simulink model "LinksVDCR1"  (R2020b)
settings: Solver=ode45  StartTime=0.0  StopTime=20  FixedStep=0.001  RelTol=1e-5  AbsTol=1e-5
undefined symbols (not defined in the file or in its folder): X, Y, Z
libraries: sm_lib x18, nesl_utility x9
settings Model: Creator=liikaneh  LastModifiedBy=humaloja
settings SolverCC: ZeroCrossAlgorithm=Adaptive  AlgebraicLoopSolver=LineSearch
settings DataIOCC: ReturnWorkspaceOutputs=off
settings DebuggingCC: ArithmeticOperatorsInVariantConditions=warning
settings SFSimCC: SimUseLocalCustomCode=off  CustomCodeUndefinedFunction=UseInterfaceOnly
settings RTWCC: RTWUseLocalCustomCode=off

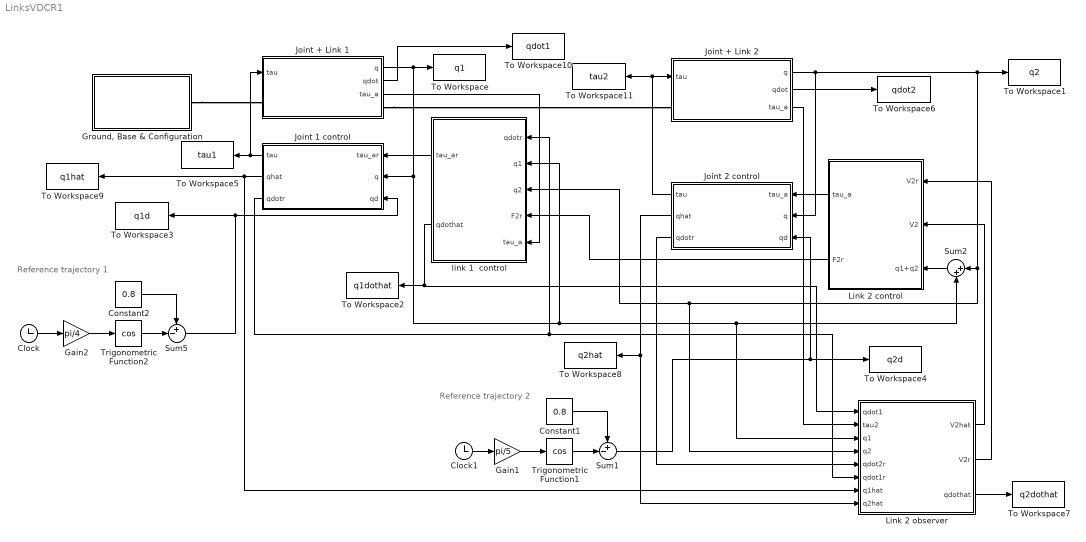
== system LinksVDCR1 ==
  note: Reference trajectory 1
  note: Reference trajectory 2
  Clock : Clock
  Clock1 : Clock
  Constant1 : Constant  Value=0.8
  Constant2 : Constant  Value=0.8
  Gain1 : Gain  Gain=pi/5
  Gain2 : Gain  Gain=pi/4
  "Ground, Base & Configuration" : Subsystem
  Joint + Link 1 : Subsystem
  Joint + Link 2 : Subsystem
  Joint 1 control : Subsystem
  Joint 2 control : Subsystem
  Link 2 control : Subsystem
  Link 2 observer : Subsystem
  Sum1 : Sum  Inputs=+-|
  Sum2 : Sum  Inputs=|++
  Sum5 : Sum  Inputs=+-|
  To Workspace : ToWorkspace  VariableName=q1  SaveFormat=Timeseries  SampleTime=-1
  To Workspace1 : ToWorkspace  VariableName=q2  SaveFormat=Timeseries  SampleTime=-1
  To Workspace10 : ToWorkspace  VariableName=qdot1  SaveFormat=Timeseries  SampleTime=-1
  To Workspace11 : ToWorkspace  VariableName=tau2  SaveFormat=Timeseries  SampleTime=-1
  To Workspace2 : ToWorkspace  VariableName=q1dothat  SaveFormat=Timeseries  SampleTime=-1
  To Workspace3 : ToWorkspace  VariableName=q1d  SaveFormat=Timeseries  SampleTime=-1
  To Workspace4 : ToWorkspace  VariableName=q2d  SaveFormat=Timeseries  SampleTime=-1
  To Workspace5 : ToWorkspace  VariableName=tau1  SaveFormat=Timeseries  SampleTime=-1
  To Workspace6 : ToWorkspace  VariableName=qdot2  SaveFormat=Timeseries  SampleTime=-1
  To Workspace7 : ToWorkspace  VariableName=q2dothat  SaveFormat=Timeseries  SampleTime=-1
  To Workspace8 : ToWorkspace  VariableName=q2hat  SaveFormat=Timeseries  SampleTime=-1
  To Workspace9 : ToWorkspace  VariableName=q1hat  SaveFormat=Timeseries  SampleTime=-1
  Trigonometric Function1 : Trigonometry  Operator=cos
  Trigonometric Function2 : Trigonometry  Operator=cos
  link 1  control : Subsystem
  wires:
  Joint + Link 1/1(q) -> To Workspace/1, link 1  control/2(q1), Link 2 observer/3(q1), Sum2/2, Joint 1 control/2(q)
  Constant1/1 -> Sum1/1
  Joint + Link 2/1(q) -> Joint 2 control/2(q), link 1  control/3(q2), Link 2 observer/4(q2), Sum2/1, To Workspace1/1
  Sum2/1 -> Link 2 control/3(q1+q2)
  Link 2 observer/1(V2hat) -> Link 2 control/2(V2)
  Link 2 observer/2(V2r) -> Link 2 control/1(V2r)
  Clock1/1 -> Gain1/1
  Gain1/1 -> Trigonometric Function1/1
  Sum5/1 -> To Workspace3/1, Joint 1 control/3(qd)
  Sum1/1 -> Joint 2 control/3(qd), To Workspace4/1
  Constant2/1 -> Sum5/1
  Gain2/1 -> Trigonometric Function2/1
  Clock/1 -> Gain2/1
  Link 2 control/1(tau_a) -> Joint 2 control/1(tau_a)
  Joint 1 control/1(tau) -> Joint + Link 1/1(tau), To Workspace5/1
  Joint + Link 2/3(tau_a) -> Link 2 observer/2(tau2)
  Joint + Link 1/3(tau_a) -> link 1  control/5(tau_a)
  Joint 1 control/2(qhat) -> To Workspace9/1, Link 2 observer/7(q1hat)
  Joint 1 control/3(qdotr) -> Link 2 observer/6(qdot1r), link 1  control/1(qdotr)
  link 1  control/1(tau_ar) -> Joint 1 control/1(tau_ar)
  Link 2 control/2(F2r) -> link 1  control/4(F2r)
  Trigonometric Function1/1 -> Sum1/2
  Trigonometric Function2/1 -> Sum5/2
  Joint 2 control/1(tau) -> Joint + Link 2/1(tau), To Workspace11/1
  Joint 2 control/2(qhat) -> Link 2 observer/8(q2hat), To Workspace8/1
  Joint 2 control/3(qdotr) -> Link 2 observer/5(qdot2r)
  Joint + Link 1/2(qdot) -> To Workspace10/1
  Joint + Link 2/2(qdot) -> To Workspace6/1
  link 1  control/2(qdothat) -> Link 2 observer/1(qdot1), To Workspace2/1
  Link 2 observer/3(qdothat) -> To Workspace7/1
  connections:
  "Ground, Base & Configuration"/RConn1 -- Joint + Link 1/LConn1
  Joint + Link 1/RConn1 -- Joint + Link 2/LConn1

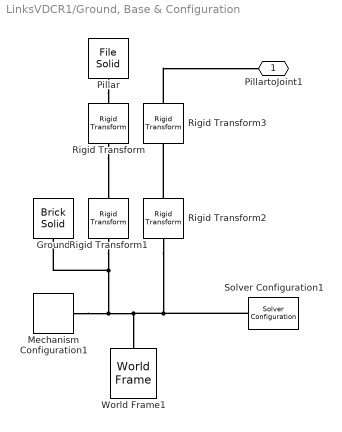
== system LinksVDCR1/Ground, Base & Configuration ==
  Ground : sm_lib/Body Elements/Brick Solid  GraphicAmbientColor=[0.15 0.15 0.15 1.0]  BasedOnType=Density  BrickDimensions=[1 1 0.05]  BrickDimensionUnits=m  CenterOfMass=[0 0 0]  CenterOfMassUnits=m  GraphicDiffuseColor=[0.2 0.2 0.2]  Density=1000  DensityUnits=kg/m^3  DoExposeReferenceFrame=on  GraphicEmissiveColor=[0.0 0.0 0.0 1.0]  ExportEntireGeometry=off  SerializedFrames=<Frames/>  MarkerShape=Sphere  MarkerSize=10  GraphicType=FromGeometry  InertiaType=CalculateFromGeometry  Mass=1  MassUnits=kg  MomentsOfInertia=[1 1 1]  MomentsOfInertiaUnits=kg*m^2  GraphicOpacity=1.0  ProductsOfInertia=[1 1 1]  ProductsOfInertiaUnits=kg*m^2  GraphicShininess=75  GraphicSpecularColor=[0.5 0.5 0.5 1.0]  GraphicVisPropType=SimpleVisualProperties
  Mechanism Configuration1 : sm_lib/Utilities/Mechanism Configuration  UniformGravity=Constant  GravityVector=[0 0 -9.80655]  GravityVectorUnits=m/s^2  GravityUnits=m/s^2  LinearizationDelta=0.002  JointModeTransitionNonlinearIterations=2
  Pillar : sm_lib/Body Elements/File Solid  ExtGeomFileName=Base.STEP  UnitType=FromFile  ExtGeomFileUnits=m  StepReaderType=OCC  ExportConvexHullGeometry=off  InertiaType=CalculateFromGeometry  Mass=1  MassUnits=kg  CenterOfMass=[0 0 0]  CenterOfMassUnits=m  MomentsOfInertia=[1 1 1]  MomentsOfInertiaUnits=kg*m^2  ProductsOfInertia=[1 1 1]  ProductsOfInertiaUnits=kg*m^2  BasedOnType=Density  Density=1000  DensityUnits=kg/m^3  DoExposeReferenceFrame=on  SerializedFrames=<Frames/>  GraphicType=FromGeometry  MarkerShape=Sphere  MarkerSize=10  GraphicVisPropType=SimpleVisualProperties  GraphicDiffuseColor=[0.2 0.2 0.2]  GraphicSpecularColor=[0.5 0.5 0.5 1.0]  GraphicAmbientColor=[0.15 0.15 0.15 1.0]  GraphicEmissiveColor=[0.0 0.0 0.0 1.0]  GraphicShininess=75  GraphicOpacity=1.0
  Rigid Transform : sm_lib/Frames and Transforms/Rigid Transform  TranslationMethod=None  TranslationStandardOffset=0  TranslationLengthUnit=m  TranslationStandardAxis=+Z  TranslationCartesianOffset=[0 0 0]  TranslationROffset=0  TranslationROffsetUnits=m  TranslationZOffset=0  TranslationZOffsetUnits=m  TranslationThetaOffset=0  TranslationThetaOffsetUnits=deg  RotationMethod=StandardAxis  RotationAngleUnits=deg  RotationStandardAxis=+Y  RotationAngle=180  RotationArbitraryAxis=[0 0 1]  FollAlignAxisA=+X  BaseAlignAxisA=+Y  FollAlignAxisB=+Y  BaseAlignAxisB=+Z  RotationSequenceAxes=FollowerAxes  RotationSequence=XYX  RotationSequenceAngles=[0 0 0]  RotationSequenceAnglesUnits=deg  RotationMatrix=[1 0 0; 0 1 0; 0 0 1]
  Rigid Transform1 : sm_lib/Frames and Transforms/Rigid Transform  TranslationMethod=None  TranslationStandardOffset=0  TranslationLengthUnit=m  TranslationStandardAxis=+Z  TranslationCartesianOffset=[0 0 0]  TranslationROffset=0  TranslationROffsetUnits=m  TranslationZOffset=0  TranslationZOffsetUnits=m  TranslationThetaOffset=0  TranslationThetaOffsetUnits=deg  RotationMethod=StandardAxis  RotationAngleUnits=deg  RotationStandardAxis=+Z  RotationAngle=90  RotationArbitraryAxis=[0 0 1]  FollAlignAxisA=+X  BaseAlignAxisA=+Y  FollAlignAxisB=+Y  BaseAlignAxisB=+Z  RotationSequenceAxes=FollowerAxes  RotationSequence=XYX  RotationSequenceAngles=[0 0 0]  RotationSequenceAnglesUnits=deg  RotationMatrix=[1 0 0; 0 1 0; 0 0 1]
  Rigid Transform2 : sm_lib/Frames and Transforms/Rigid Transform  TranslationMethod=StandardAxis  TranslationStandardOffset=0.470  TranslationLengthUnit=m  TranslationStandardAxis=+Z  TranslationCartesianOffset=[0 0 0]  TranslationROffset=0  TranslationROffsetUnits=m  TranslationZOffset=0  TranslationZOffsetUnits=m  TranslationThetaOffset=0  TranslationThetaOffsetUnits=deg  RotationMethod=None  RotationAngleUnits=deg  RotationStandardAxis=+Z  RotationAngle=0.0  RotationArbitraryAxis=[0 0 1]  FollAlignAxisA=+X  BaseAlignAxisA=+Y  FollAlignAxisB=+Y  BaseAlignAxisB=+Z  RotationSequenceAxes=FollowerAxes  RotationSequence=XYX  RotationSequenceAngles=[0 0 0]  RotationSequenceAnglesUnits=deg  RotationMatrix=[1 0 0; 0 1 0; 0 0 1]
  Rigid Transform3 : sm_lib/Frames and Transforms/Rigid Transform  TranslationMethod=None  TranslationStandardOffset=0  TranslationLengthUnit=m  TranslationStandardAxis=+Z  TranslationCartesianOffset=[0 0 0]  TranslationROffset=0  TranslationROffsetUnits=m  TranslationZOffset=0  TranslationZOffsetUnits=m  TranslationThetaOffset=0  TranslationThetaOffsetUnits=deg  RotationMethod=StandardAxis  RotationAngleUnits=deg  RotationStandardAxis=+X  RotationAngle=90  RotationArbitraryAxis=[0 0 1]  FollAlignAxisA=+X  BaseAlignAxisA=+Y  FollAlignAxisB=+Y  BaseAlignAxisB=+Z  RotationSequenceAxes=FollowerAxes  RotationSequence=XYX  RotationSequenceAngles=[0 0 0]  RotationSequenceAnglesUnits=deg  RotationMatrix=[1 0 0; 0 1 0; 0 0 1]
  Solver Configuration1 : nesl_utility/Solver Configuration  PhysicalDomain=network_engine_domain  SubClassName=solver  LeftPortType=input  RightPortType=generic  Tones=[]  Harmonics=[]  SimulateNoise=off  Profile=off  UseLocalSampling=off  EnableSwitchedLinearOptims=on  FrequencyDomain=off  UseCCode=off  RelTol=0.001  AbsTol=1e-06  MinStep=1e-09  ToWorkspace=off  RevertToSquareIcSolve=off  NumHomotopyIterations=100  PhasorMode=off  PhasorModeNumHarmonics=1  DoDC=off  ResidualTolerance=1e-9  UseLocalSolver=off  LocalSolverChoice=NE_BACKWARD_EULER_ADVANCER  LocalSolverSampleTime=0.002  DoFixedCost=off  MaxNonlinIter=3  MaxModeIter=2  ComputeImpulses=off  ImpulseIterations=2  LinearAlgebra=Sparse  EquationFormulation=NE_TIME_EF  DelaysMemoryBudget=1024  AutomaticFiltering=on  FilteringTimeConstant=0.002  PartitionStorageMethod=AS_NEEDED  PartitionMemoryBudget=1024  PartitionMethod=FAST
  World Frame1 : sm_lib/Frames and Transforms/World Frame
  PillartoJoint1 : PMIOPort  Side=Right
  connections:
  Solver Configuration1/RConn1 -- Rigid Transform2/LConn1 -- Ground/RConn1 -- Rigid Transform1/LConn1 -- Mechanism Configuration1/RConn1 -- World Frame1/RConn1
  Rigid Transform3/RConn1 -- PillartoJoint1/RConn1
  Pillar/RConn1 -- Rigid Transform/RConn1
  Rigid Transform2/RConn1 -- Rigid Transform3/LConn1
  Rigid Transform/LConn1 -- Rigid Transform1/RConn1

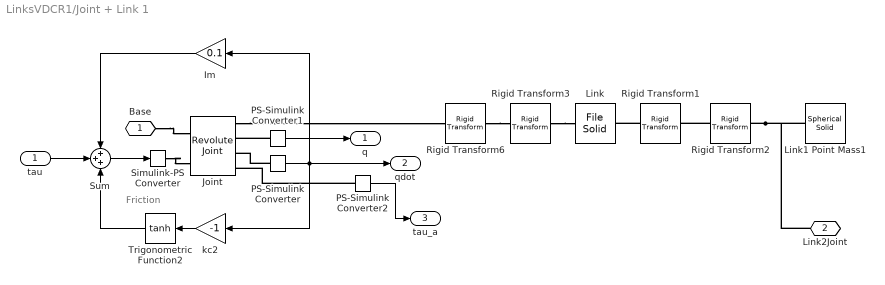
== system LinksVDCR1/Joint + Link 1 ==
  note: Friction
  tau : Inport
  Im : Gain  Gain=0.1
  Joint : sm_lib/Joints/Revolute Joint  JointMode=Normal  SenseConstraintForce=off  SenseConstraintForceX=off  SenseConstraintForceY=off  SenseConstraintForceZ=off  SenseConstraintTorque=off  SenseConstraintTorqueX=off  SenseConstraintTorqueY=off  SenseConstraintTorqueZ=off  SenseTotalForce=off  SenseTotalForceX=off  SenseTotalForceY=off  SenseTotalForceZ=off  SenseTotalTorque=off  SenseTotalTorqueX=off  SenseTotalTorqueY=off  SenseTotalTorqueZ=off  CompositeWrenchDir=FollowerOnBase  CompositeWrenchFrame=BaseFrame  EquilibriumPosition=0  EquilibriumPositionUnits=deg  SpringStiffness=0  SpringStiffnessUnits=N*m/deg  DampingCoefficient=0  DampingCoefficientUnits=N*m/(deg/s)  TorqueActuationMode=InputTorque  MotionActuationMode=ComputedMotion  SensePosition=on  SenseVelocity=on  SenseAcceleration=off  SenseTorqueForce=on  SenseLowerLimitTorqueForce=off  SenseUpperLimitTorqueForce=off  LowerLimitSpecify=off  LowerLimitBound=0  LowerLimitBoundUnits=deg  LowerLimitStiffness=1e4  LowerLimitStiffnessUnits=N*m/deg  LowerLimitDamping=10  LowerLimitDampingUnits=N*m/(deg/s)  LowerLimitTransitionRegionWidth=0.1  LowerLimitTransitionRegionWidthUnits=deg  UpperLimitSpecify=off  UpperLimitBound=0  UpperLimitBoundUnits=deg  UpperLimitStiffness=1e4  UpperLimitStiffnessUnits=N*m/deg  UpperLimitDamping=10  UpperLimitDampingUnits=N*m/(deg/s)  UpperLimitTransitionRegionWidth=0.1  UpperLimitTransitionRegionWidthUnits=deg  PositionTargetSpecify=on  PositionTargetPriority=High  PositionTargetValue=0  PositionTargetValueUnits=deg  VelocityTargetSpecify=off  VelocityTargetPriority=High  VelocityTargetValue=0  VelocityTargetValueUnits=deg/s
  Link : sm_lib/Body Elements/File Solid  ExtGeomFileName=link1.STEP  UnitType=FromFile  ExtGeomFileUnits=m  StepReaderType=OCC  ExportConvexHullGeometry=off  InertiaType=CalculateFromGeometry  Mass=0  MassUnits=kg  CenterOfMass=[0 0 0]  CenterOfMassUnits=m  MomentsOfInertia=[1 1 1]  MomentsOfInertiaUnits=kg*m^2  ProductsOfInertia=[1 1 1]  ProductsOfInertiaUnits=kg*m^2  BasedOnType=Mass  Density=1000  DensityUnits=kg/m^3  DoExposeReferenceFrame=on  SerializedFrames=<Frames><Frame><Id>Frame1</Id><Value><Name>F1</Name><Origin><Source>GeometricFeature</Source><FeatureName>circular curve 61</FeatureName></Origin><PrimaryAxis><DefinedDirection>+Z</DefinedDirection><Source>ReferenceFrame</Source><SourceDirection>+Z</SourceDirection><FeatureName></FeatureName></PrimaryAxis><SecondaryAxis><DefinedDirection>+X</DefinedDirection><Source>ReferenceFrame</Source><SourceDirection>+X</SourceDirection><FeatureName></FeatureName></SecondaryAxis></Value></Frame></Frames>  GraphicType=FromGeometry  MarkerShape=Sphere  MarkerSize=10  GraphicVisPropType=SimpleVisualProperties  GraphicDiffuseColor=[0.5 0.5 0.5]  GraphicSpecularColor=[0.5 0.5 0.5 1.0]  GraphicAmbientColor=[0.15 0.15 0.15 1.0]  GraphicEmissiveColor=[0.0 0.0 0.0 1.0]  GraphicShininess=75  GraphicOpacity=1.0
  Link1 Point Mass1 : sm_lib/Body Elements/Spherical Solid  GraphicAmbientColor=[0.15 0.15 0.15 1.0]  BasedOnType=Mass  CenterOfMass=[0 0 0]  CenterOfMassUnits=m  GraphicDiffuseColor=[0.0 0.0 0.0]  Density=1000  DensityUnits=kg/m^3  DoExposeReferenceFrame=on  GraphicEmissiveColor=[0.0 0.0 0.0 1.0]  ExportEntireGeometry=off  SerializedExposedGeometries=<ExposedGeometries/>  SerializedFrames=<Frames/>  MarkerShape=Sphere  MarkerSize=10  GraphicType=FromGeometry  InertiaType=PointMass  Mass=1  MassUnits=kg  MomentsOfInertia=[1 1 1]  MomentsOfInertiaUnits=kg*m^2  GraphicOpacity=1.0  ProductsOfInertia=[1 1 1]  ProductsOfInertiaUnits=kg*m^2  GraphicShininess=75  GraphicSpecularColor=[0.5 0.5 0.5 1.0]  SphereRadius=0.10  SphereRadiusUnits=m  GraphicVisPropType=SimpleVisualProperties
  PS-Simulink Converter : nesl_utility/PS-Simulink Converter  PhysicalDomain=network_engine_domain  SubClassName=ps_output  LeftPortType=input  RightPortType=output  PseudoPeriodic=off  Frequencies=[]  Unit=inherit  AffineConversion=off
  PS-Simulink Converter1 : nesl_utility/PS-Simulink Converter  PhysicalDomain=network_engine_domain  SubClassName=ps_output  LeftPortType=input  RightPortType=output  PseudoPeriodic=off  Frequencies=[]  Unit=inherit  AffineConversion=off
  PS-Simulink Converter2 : nesl_utility/PS-Simulink Converter  PhysicalDomain=network_engine_domain  SubClassName=ps_output  LeftPortType=input  RightPortType=output  PseudoPeriodic=off  Frequencies=[]  Unit=inherit  AffineConversion=off
  Rigid Transform1 : sm_lib/Frames and Transforms/Rigid Transform  TranslationMethod=None  TranslationStandardOffset=0  TranslationLengthUnit=m  TranslationStandardAxis=+Z  TranslationCartesianOffset=[0 0 0]  TranslationROffset=0  TranslationROffsetUnits=m  TranslationZOffset=0  TranslationZOffsetUnits=m  TranslationThetaOffset=0  TranslationThetaOffsetUnits=deg  RotationMethod=StandardAxis  RotationAngleUnits=deg  RotationStandardAxis=-Y  RotationAngle=90  RotationArbitraryAxis=[0 0 1]  FollAlignAxisA=+X  BaseAlignAxisA=+Y  FollAlignAxisB=+Y  BaseAlignAxisB=+Z  RotationSequenceAxes=FollowerAxes  RotationSequence=XYX  RotationSequenceAngles=[0 0 0]  RotationSequenceAnglesUnits=deg  RotationMatrix=[1 0 0; 0 1 0; 0 0 1]
  Rigid Transform2 : sm_lib/Frames and Transforms/Rigid Transform  TranslationMethod=StandardAxis  TranslationStandardOffset=0.035  TranslationLengthUnit=m  TranslationStandardAxis=+Z  TranslationCartesianOffset=[0 0 0]  TranslationROffset=0  TranslationROffsetUnits=m  TranslationZOffset=0  TranslationZOffsetUnits=m  TranslationThetaOffset=0  TranslationThetaOffsetUnits=deg  RotationMethod=None  RotationAngleUnits=deg  RotationStandardAxis=-Y  RotationAngle=90  RotationArbitraryAxis=[0 0 1]  FollAlignAxisA=+X  BaseAlignAxisA=+Y  FollAlignAxisB=+Y  BaseAlignAxisB=+Z  RotationSequenceAxes=FollowerAxes  RotationSequence=XYX  RotationSequenceAngles=[0 0 0]  RotationSequenceAnglesUnits=deg  RotationMatrix=[1 0 0; 0 1 0; 0 0 1]
  Rigid Transform3 : sm_lib/Frames and Transforms/Rigid Transform  TranslationMethod=StandardAxis  TranslationStandardOffset=0.05  TranslationLengthUnit=m  TranslationStandardAxis=+Z  TranslationCartesianOffset=[0 0 0]  TranslationROffset=0  TranslationROffsetUnits=m  TranslationZOffset=0  TranslationZOffsetUnits=m  TranslationThetaOffset=0  TranslationThetaOffsetUnits=deg  RotationMethod=None  RotationAngleUnits=deg  RotationStandardAxis=+Z  RotationAngle=0.0  RotationArbitraryAxis=[0 0 1]  FollAlignAxisA=+X  BaseAlignAxisA=+Y  FollAlignAxisB=+Y  BaseAlignAxisB=+Z  RotationSequenceAxes=FollowerAxes  RotationSequence=XYX  RotationSequenceAngles=[0 0 0]  RotationSequenceAnglesUnits=deg  RotationMatrix=[1 0 0; 0 1 0; 0 0 1]
  Rigid Transform6 : sm_lib/Frames and Transforms/Rigid Transform  TranslationMethod=None  TranslationStandardOffset=0  TranslationLengthUnit=m  TranslationStandardAxis=+Z  TranslationCartesianOffset=[0 0 0]  TranslationROffset=0  TranslationROffsetUnits=m  TranslationZOffset=0  TranslationZOffsetUnits=m  TranslationThetaOffset=0  TranslationThetaOffsetUnits=deg  RotationMethod=StandardAxis  RotationAngleUnits=deg  RotationStandardAxis=-Y  RotationAngle=90  RotationArbitraryAxis=[0 0 1]  FollAlignAxisA=+X  BaseAlignAxisA=+Y  FollAlignAxisB=+Y  BaseAlignAxisB=+Z  RotationSequenceAxes=FollowerAxes  RotationSequence=XYX  RotationSequenceAngles=[0 0 0]  RotationSequenceAnglesUnits=deg  RotationMatrix=[1 0 0; 0 1 0; 0 0 1]
  Simulink-PS Converter : nesl_utility/Simulink-PS Converter  PhysicalDomain=network_engine_domain  SubClassName=ps_input  LeftPortType=input  RightPortType=output  PseudoPeriodic=off  Frequencies=[]  NoiseDistribution=none  NoiseParameters=[]  Unit=1  AffineConversion=off  FilteringAndDerivatives=provide  SimscapeFilterOrder=1  InputFilterTimeConstant=0.001  UdotUserProvided=0
  Sum : Sum  Inputs=+++
  Trigonometric Function2 : Trigonometry  Operator=tanh
  kc2 : Gain  Gain=-1
  Base : PMIOPort  Side=Left
  Link2Joint : PMIOPort  Port=2  Side=Right
  q : Outport
  qdot : Outport  Port=2
  tau_a : Outport  Port=3
  wires:
  Trigonometric Function2/1 -> Sum/3
  kc2/1 -> Trigonometric Function2/1
  tau/1 -> Sum/2
  Sum/1 -> Simulink-PS Converter/1
  Im/1 -> Sum/1
  PS-Simulink Converter/1 -> Im/1, kc2/1, qdot/1
  PS-Simulink Converter1/1 -> q/1
  PS-Simulink Converter2/1 -> tau_a/1
  connections:
  Base/RConn1 -- Joint/LConn1
  Simulink-PS Converter/RConn1 -- Joint/LConn2
  PS-Simulink Converter/LConn1 -- Joint/RConn3
  PS-Simulink Converter1/LConn1 -- Joint/RConn2
  Rigid Transform2/RConn1 -- Link2Joint/RConn1 -- Link1 Point Mass1/RConn1
  Rigid Transform1/RConn1 -- Link/LConn1
  Rigid Transform6/RConn1 -- Rigid Transform3/RConn1
  Rigid Transform3/LConn1 -- Link/RConn1
  Rigid Transform2/LConn1 -- Rigid Transform1/LConn1
  Joint/RConn1 -- Rigid Transform6/LConn1
  PS-Simulink Converter2/LConn1 -- Joint/RConn4

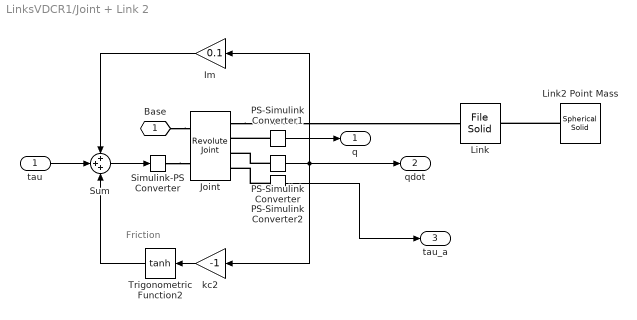
== system LinksVDCR1/Joint + Link 2 ==
  note: Friction
  tau : Inport
  Im : Gain  Gain=0.1
  Joint : sm_lib/Joints/Revolute Joint  JointMode=Normal  SenseConstraintForce=off  SenseConstraintForceX=off  SenseConstraintForceY=off  SenseConstraintForceZ=off  SenseConstraintTorque=off  SenseConstraintTorqueX=off  SenseConstraintTorqueY=off  SenseConstraintTorqueZ=off  SenseTotalForce=off  SenseTotalForceX=off  SenseTotalForceY=off  SenseTotalForceZ=off  SenseTotalTorque=off  SenseTotalTorqueX=off  SenseTotalTorqueY=off  SenseTotalTorqueZ=off  CompositeWrenchDir=FollowerOnBase  CompositeWrenchFrame=BaseFrame  EquilibriumPosition=0  EquilibriumPositionUnits=deg  SpringStiffness=0  SpringStiffnessUnits=N*m/deg  DampingCoefficient=0  DampingCoefficientUnits=N*m/(deg/s)  TorqueActuationMode=InputTorque  MotionActuationMode=ComputedMotion  SensePosition=on  SenseVelocity=on  SenseAcceleration=off  SenseTorqueForce=on  SenseLowerLimitTorqueForce=off  SenseUpperLimitTorqueForce=off  LowerLimitSpecify=off  LowerLimitBound=0  LowerLimitBoundUnits=deg  LowerLimitStiffness=1e4  LowerLimitStiffnessUnits=N*m/deg  LowerLimitDamping=10  LowerLimitDampingUnits=N*m/(deg/s)  LowerLimitTransitionRegionWidth=0.1  LowerLimitTransitionRegionWidthUnits=deg  UpperLimitSpecify=off  UpperLimitBound=0  UpperLimitBoundUnits=deg  UpperLimitStiffness=1e4  UpperLimitStiffnessUnits=N*m/deg  UpperLimitDamping=10  UpperLimitDampingUnits=N*m/(deg/s)  UpperLimitTransitionRegionWidth=0.1  UpperLimitTransitionRegionWidthUnits=deg  PositionTargetSpecify=on  PositionTargetPriority=High  PositionTargetValue=0  PositionTargetValueUnits=deg  VelocityTargetSpecify=off  VelocityTargetPriority=High  VelocityTargetValue=0  VelocityTargetValueUnits=deg/s
  Link : sm_lib/Body Elements/File Solid  ExtGeomFileName=link2.STEP  UnitType=FromFile  ExtGeomFileUnits=m  StepReaderType=OCC  ExportConvexHullGeometry=off  InertiaType=CalculateFromGeometry  Mass=0  MassUnits=kg  CenterOfMass=[0 0 0]  CenterOfMassUnits=m  MomentsOfInertia=[1 1 1]  MomentsOfInertiaUnits=kg*m^2  ProductsOfInertia=[1 1 1]  ProductsOfInertiaUnits=kg*m^2  BasedOnType=Mass  Density=1000  DensityUnits=kg/m^3  DoExposeReferenceFrame=on  SerializedFrames=<Frames><Frame><Id>Frame1</Id><Value><Name>F1</Name><Origin><Source>GeometricFeature</Source><FeatureName>planar surface 7</FeatureName></Origin><PrimaryAxis><DefinedDirection>+Z</DefinedDirection><Source>ReferenceFrame</Source><SourceDirection>+Z</SourceDirection><FeatureName></FeatureName></PrimaryAxis><SecondaryAxis><DefinedDirection>+X</DefinedDirection><Source>ReferenceFrame</Source><SourceDirection>+X</SourceDirection><FeatureName></FeatureName></SecondaryAxis></Value></Frame></Frames>  GraphicType=FromGeometry  MarkerShape=Sphere  MarkerSize=10  GraphicVisPropType=SimpleVisualProperties  GraphicDiffuseColor=[0.5 0.5 0.5]  GraphicSpecularColor=[0.5 0.5 0.5 1.0]  GraphicAmbientColor=[0.15 0.15 0.15 1.0]  GraphicEmissiveColor=[0.0 0.0 0.0 1.0]  GraphicShininess=75  GraphicOpacity=1.0
  Link2 Point Mass : sm_lib/Body Elements/Spherical Solid  GraphicAmbientColor=[0.15 0.15 0.15 1.0]  BasedOnType=Mass  CenterOfMass=[0 0 0]  CenterOfMassUnits=m  GraphicDiffuseColor=[0.0 0.0 0.0]  Density=1000  DensityUnits=kg/m^3  DoExposeReferenceFrame=on  GraphicEmissiveColor=[0.0 0.0 0.0 1.0]  ExportEntireGeometry=off  SerializedExposedGeometries=<ExposedGeometries/>  SerializedFrames=<Frames/>  MarkerShape=Sphere  MarkerSize=10  GraphicType=FromGeometry  InertiaType=PointMass  Mass=1  MassUnits=kg  MomentsOfInertia=[1 1 1]  MomentsOfInertiaUnits=kg*m^2  GraphicOpacity=1.0  ProductsOfInertia=[1 1 1]  ProductsOfInertiaUnits=kg*m^2  GraphicShininess=75  GraphicSpecularColor=[0.5 0.5 0.5 1.0]  SphereRadius=0.10  SphereRadiusUnits=m  GraphicVisPropType=SimpleVisualProperties
  PS-Simulink Converter : nesl_utility/PS-Simulink Converter  PhysicalDomain=network_engine_domain  SubClassName=ps_output  LeftPortType=input  RightPortType=output  PseudoPeriodic=off  Frequencies=[]  Unit=inherit  AffineConversion=off
  PS-Simulink Converter1 : nesl_utility/PS-Simulink Converter  PhysicalDomain=network_engine_domain  SubClassName=ps_output  LeftPortType=input  RightPortType=output  PseudoPeriodic=off  Frequencies=[]  Unit=inherit  AffineConversion=off
  PS-Simulink Converter2 : nesl_utility/PS-Simulink Converter  PhysicalDomain=network_engine_domain  SubClassName=ps_output  LeftPortType=input  RightPortType=output  PseudoPeriodic=off  Frequencies=[]  Unit=inherit  AffineConversion=off
  Simulink-PS Converter : nesl_utility/Simulink-PS Converter  PhysicalDomain=network_engine_domain  SubClassName=ps_input  LeftPortType=input  RightPortType=output  PseudoPeriodic=off  Frequencies=[]  NoiseDistribution=none  NoiseParameters=[]  Unit=1  AffineConversion=off  FilteringAndDerivatives=provide  SimscapeFilterOrder=1  InputFilterTimeConstant=0.001  UdotUserProvided=0
  Sum : Sum  Inputs=+++
  Trigonometric Function2 : Trigonometry  Operator=tanh
  kc2 : Gain  Gain=-1
  Base : PMIOPort  Side=Left
  q : Outport
  qdot : Outport  Port=2
  tau_a : Outport  Port=3
  wires:
  Trigonometric Function2/1 -> Sum/3
  kc2/1 -> Trigonometric Function2/1
  tau/1 -> Sum/2
  Sum/1 -> Simulink-PS Converter/1
  Im/1 -> Sum/1
  PS-Simulink Converter/1 -> Im/1, qdot/1, kc2/1
  PS-Simulink Converter1/1 -> q/1
  PS-Simulink Converter2/1 -> tau_a/1
  connections:
  Base/RConn1 -- Joint/LConn1
  Simulink-PS Converter/RConn1 -- Joint/LConn2
  PS-Simulink Converter/LConn1 -- Joint/RConn3
  PS-Simulink Converter1/LConn1 -- Joint/RConn2
  Link2 Point Mass/RConn1 -- Link/LConn1
  Joint/RConn1 -- Link/RConn1
  PS-Simulink Converter2/LConn1 -- Joint/RConn4

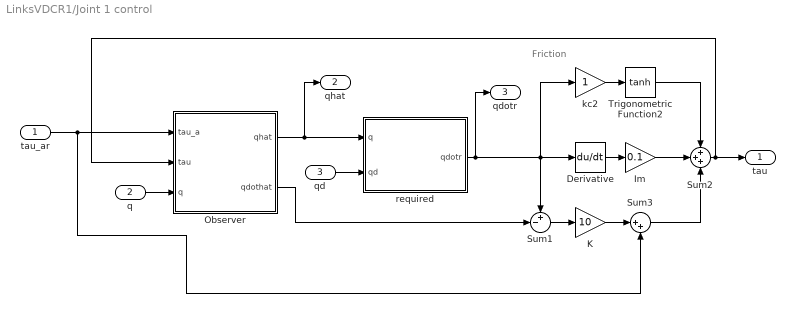
== system LinksVDCR1/Joint 1 control ==
  note: Friction
  tau_ar : Inport
  q : Inport  Port=2
  qd : Inport  Port=3
  Derivative : Derivative
  Im : Gain  Gain=0.1
  K : Gain  Gain=10
  Observer : Subsystem
  Sum1 : Sum  Inputs=+-|
  Sum2 : Sum  Inputs=+++
  Sum3 : Sum  Inputs=|++
  Trigonometric Function2 : Trigonometry  Operator=tanh
  kc2 : Gain
  required : Subsystem
  tau : Outport
  qhat : Outport  Port=2
  qdotr : Outport  Port=3
  wires:
  kc2/1 -> Trigonometric Function2/1
  q/1 -> Observer/3(q)
  Observer/1(qhat) -> qhat/1, required/1(q)
  qd/1 -> required/2(qd)
  Sum1/1 -> K/1
  Derivative/1 -> Im/1
  Sum2/1 -> tau/1, Observer/2(tau)
  Im/1 -> Sum2/2
  Observer/2(qdothat) -> Sum1/2
  required/1(qdotr) -> qdotr/1, kc2/1, Derivative/1, Sum1/1
  Trigonometric Function2/1 -> Sum2/1
  K/1 -> Sum3/1
  Sum3/1 -> Sum2/3
  tau_ar/1 -> Sum3/2, Observer/1(tau_a)

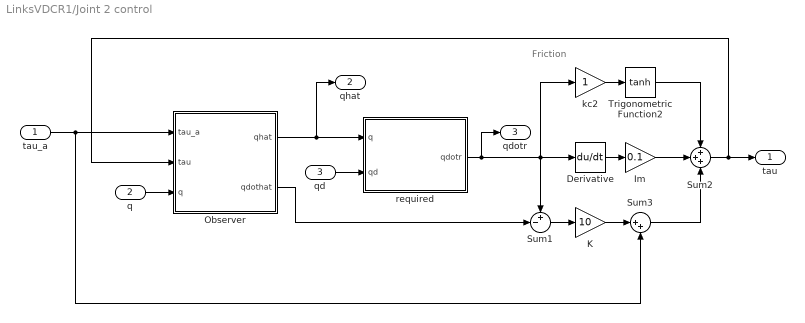
== system LinksVDCR1/Joint 2 control ==
  note: Friction
  tau_a : Inport
  q : Inport  Port=2
  qd : Inport  Port=3
  Derivative : Derivative
  Im : Gain  Gain=0.1
  K : Gain  Gain=10
  Observer : Subsystem
  Sum1 : Sum  Inputs=+-|
  Sum2 : Sum  Inputs=+++
  Sum3 : Sum  Inputs=|++
  Trigonometric Function2 : Trigonometry  Operator=tanh
  kc2 : Gain
  required : Subsystem
  tau : Outport
  qhat : Outport  Port=2
  qdotr : Outport  Port=3
  wires:
  kc2/1 -> Trigonometric Function2/1
  tau_a/1 -> Sum3/2, Observer/1(tau_a)
  q/1 -> Observer/3(q)
  Observer/1(qhat) -> qhat/1, required/1(q)
  qd/1 -> required/2(qd)
  Sum1/1 -> K/1
  Derivative/1 -> Im/1
  Sum2/1 -> tau/1, Observer/2(tau)
  Im/1 -> Sum2/2
  Observer/2(qdothat) -> Sum1/2
  required/1(qdotr) -> qdotr/1, kc2/1, Derivative/1, Sum1/1
  Trigonometric Function2/1 -> Sum2/1
  K/1 -> Sum3/1
  Sum3/1 -> Sum2/3

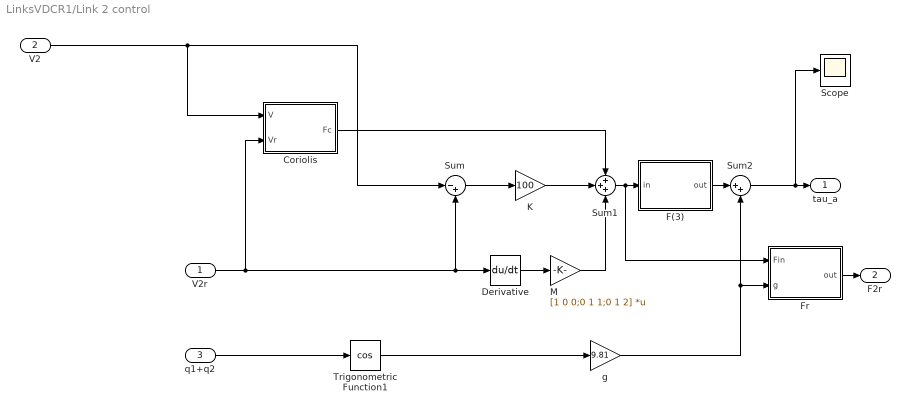
== system LinksVDCR1/Link 2 control ==
  V2r : Inport
  V2 : Inport  Port=2
  q1+q2 : Inport  Port=3
  Coriolis : MATLAB Function  TreatAsAtomicUnit=on
  Derivative : Derivative
  F(3) : MATLAB Function  TreatAsAtomicUnit=on
  Fr : MATLAB Function  TreatAsAtomicUnit=on
  K : Gain  Gain=100
  M : Gain  Gain=[1 0 0;0 1 1;0 1 2]  Multiplication=Matrix(K*u) (u vector)
  Scope : Scope
  Sum : Sum  Inputs=|-+
  Sum1 : Sum  Inputs=+++
  Sum2 : Sum  Inputs=|++
  Trigonometric Function1 : Trigonometry  Operator=cos
  g : Gain  Gain=9.81
  tau_a : Outport  VectorParamsAs1DForOutWhenUnconnected=off
  F2r : Outport  Port=2  VectorParamsAs1DForOutWhenUnconnected=off
  wires:
  V2r/1 -> Derivative/1, Sum/2, Coriolis/2(Vr)
  Sum/1 -> K/1
  g/1 -> Sum2/2, Fr/2(g)
  Trigonometric Function1/1 -> g/1
  K/1 -> Sum1/2
  Coriolis/1(Fc) -> Sum1/1
  V2/1 -> Coriolis/1(V), Sum/1
  q1+q2/1 -> Trigonometric Function1/1
  Sum1/1 -> Fr/1(Fin), F(3)/1(in)
  Derivative/1 -> M/1
  M/1 -> Sum1/3
  Fr/1(out) -> F2r/1
  Sum2/1 -> Scope/1, tau_a/1
  F(3)/1(out) -> Sum2/1

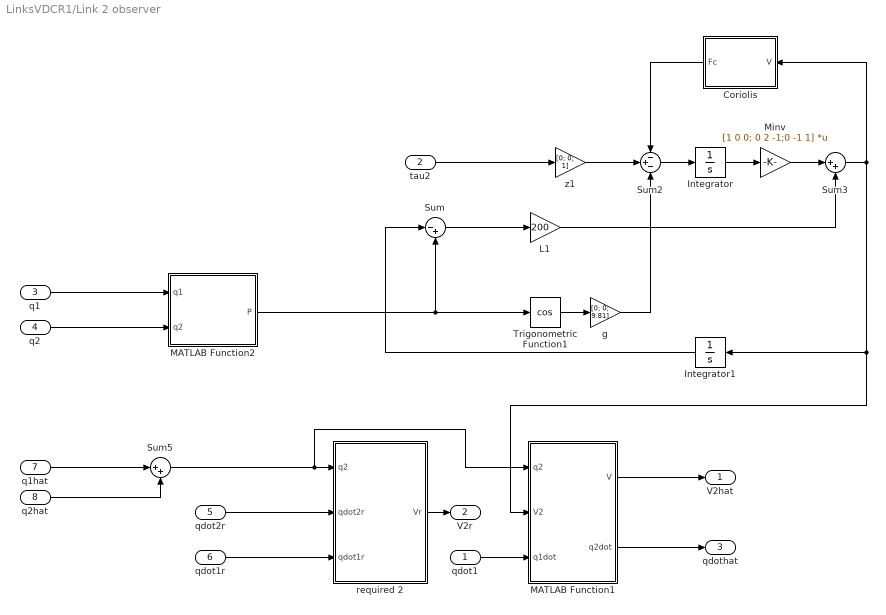
== system LinksVDCR1/Link 2 observer ==
  qdot1 : Inport
  tau2 : Inport  Port=2
  q1 : Inport  Port=3
  q2 : Inport  Port=4
  qdot2r : Inport  Port=5
  qdot1r : Inport  Port=6
  q1hat : Inport  Port=7
  q2hat : Inport  Port=8
  Coriolis : MATLAB Function  TreatAsAtomicUnit=on
  Integrator : Integrator
  Integrator1 : Integrator
  L1 : Gain  Gain=200
  MATLAB Function1 : MATLAB Function  TreatAsAtomicUnit=on
  MATLAB Function2 : MATLAB Function  TreatAsAtomicUnit=on
  Minv : Gain  Gain=[1 0 0; 0 2 -1;0 -1 1]  Multiplication=Matrix(K*u) (u vector)
  Sum : Sum  Inputs=|-+
  Sum2 : Sum  Inputs=-+-
  Sum3 : Sum  Inputs=|++
  Sum5 : Sum  Inputs=|++
  Trigonometric Function1 : Trigonometry  Operator=cos
  g : Gain  Gain=[0; 0; 9.81]
  required 2 : MATLAB Function  TreatAsAtomicUnit=on
  z1 : Gain  Gain=[0; 0; 1]
  V2hat : Outport  VectorParamsAs1DForOutWhenUnconnected=off
  V2r : Outport  Port=2  VectorParamsAs1DForOutWhenUnconnected=off
  qdothat : Outport  Port=3  VectorParamsAs1DForOutWhenUnconnected=off
  wires:
  Sum/1 -> L1/1
  Trigonometric Function1/1 -> g/1
  Sum2/1 -> Integrator/1
  L1/1 -> Sum3/2
  Integrator1/1 -> Sum/1
  Integrator/1 -> Minv/1
  Minv/1 -> Sum3/1
  qdot2r/1 -> required 2/2(qdot2r)
  q2/1 -> MATLAB Function2/2(q2)
  q1/1 -> MATLAB Function2/1(q1)
  MATLAB Function2/1(P) -> Sum/2, Trigonometric Function1/1
  g/1 -> Sum2/3
  tau2/1 -> z1/1
  z1/1 -> Sum2/2
  Coriolis/1(Fc) -> Sum2/1
  required 2/1(Vr) -> V2r/1
  Sum3/1 -> Coriolis/1(V), MATLAB Function1/2(V2), Integrator1/1
  qdot1/1 -> MATLAB Function1/3(q1dot)
  qdot1r/1 -> required 2/3(qdot1r)
  q2hat/1 -> Sum5/2
  Sum5/1 -> required 2/1(q2), MATLAB Function1/1(q2)
  q1hat/1 -> Sum5/1
  MATLAB Function1/2(q2dot) -> qdothat/1
  MATLAB Function1/1(V) -> V2hat/1

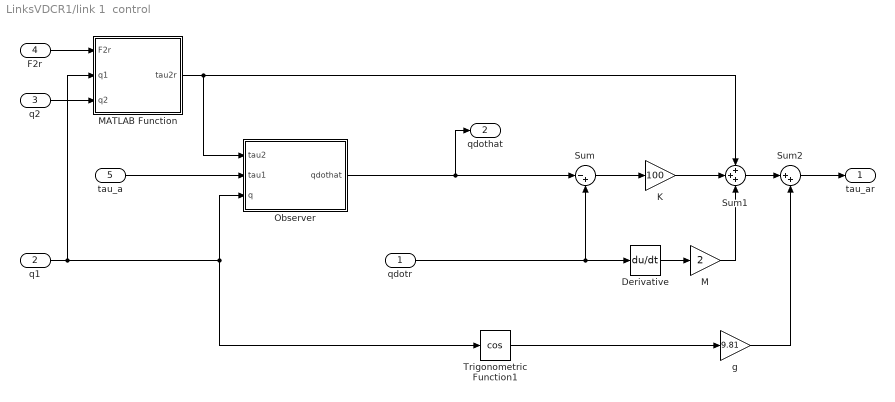
== system LinksVDCR1/link 1  control ==
  qdotr : Inport
  q1 : Inport  Port=2
  q2 : Inport  Port=3
  F2r : Inport  Port=4
  tau_a : Inport  Port=5
  Derivative : Derivative
  K : Gain  Gain=100
  M : Gain  Gain=2
  MATLAB Function : MATLAB Function  TreatAsAtomicUnit=on
  Observer : Subsystem
  Sum : Sum  Inputs=|-+
  Sum1 : Sum  Inputs=+++
  Sum2 : Sum  Inputs=|++
  Trigonometric Function1 : Trigonometry  Operator=cos
  g : Gain  Gain=9.81
  tau_ar : Outport  VectorParamsAs1DForOutWhenUnconnected=off
  qdothat : Outport  Port=2  VectorParamsAs1DForOutWhenUnconnected=off
  wires:
  qdotr/1 -> Derivative/1, Sum/2
  Sum/1 -> K/1
  g/1 -> Sum2/2
  q1/1 -> MATLAB Function/2(q1), Observer/3(q), Trigonometric Function1/1
  K/1 -> Sum1/2
  MATLAB Function/1(tau2r) -> Observer/1(tau2), Sum1/1
  Trigonometric Function1/1 -> g/1
  Derivative/1 -> M/1
  M/1 -> Sum1/3
  Observer/1(qdothat) -> qdothat/1, Sum/1
  F2r/1 -> MATLAB Function/1(F2r)
  q2/1 -> MATLAB Function/3(q2)
  Sum2/1 -> tau_ar/1
  Sum1/1 -> Sum2/1
  tau_a/1 -> Observer/2(tau1)

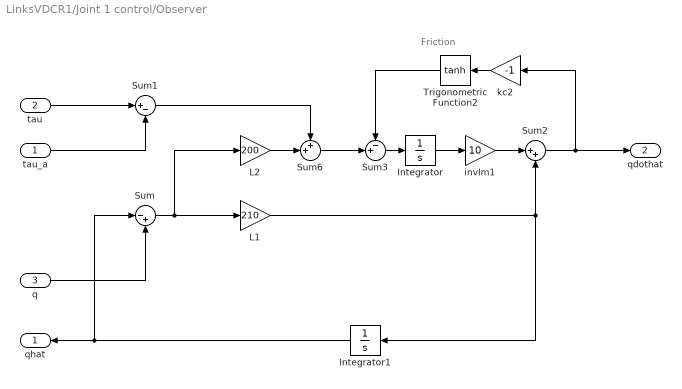
== system LinksVDCR1/Joint 1 control/Observer ==
  note: Friction
  tau_a : Inport
  tau : Inport  Port=2
  q : Inport  Port=3
  Integrator : Integrator
  Integrator1 : Integrator
  L1 : Gain  Gain=210
  L2 : Gain  Gain=200
  Sum : Sum  Inputs=|-+
  Sum1 : Sum  Inputs=|+-
  Sum2 : Sum  Inputs=|++
  Sum3 : Sum  Inputs=-+|
  Sum6 : Sum  Inputs=++|
  Trigonometric Function2 : Trigonometry  Operator=tanh
  invIm1 : Gain  Gain=10
  kc2 : Gain  Gain=-1
  qhat : Outport  VectorParamsAs1DForOutWhenUnconnected=off
  qdothat : Outport  Port=2  VectorParamsAs1DForOutWhenUnconnected=off
  wires:
  tau_a/1 -> Sum1/2
  tau/1 -> Sum1/1
  Sum/1 -> L2/1, L1/1
  q/1 -> Sum/2
  Sum1/1 -> Sum6/1
  L2/1 -> Sum6/2
  Integrator1/1 -> Sum/1, qhat/1
  L1/1 -> Integrator1/1, Sum2/2
  Sum6/1 -> Sum3/2
  kc2/1 -> Trigonometric Function2/1
  Trigonometric Function2/1 -> Sum3/1
  Sum3/1 -> Integrator/1
  Integrator/1 -> invIm1/1
  invIm1/1 -> Sum2/1
  Sum2/1 -> kc2/1, qdothat/1

== system LinksVDCR1/Joint 1 control/required ==
  q : Inport
  qd : Inport  Port=2
  Derivative : Derivative
  Sum : Sum  Inputs=+-|
  Sum1 : Sum  Inputs=++|
  lambda : Gain  Gain=10
  qdotr : Outport  VectorParamsAs1DForOutWhenUnconnected=off
  wires:
  qd/1 -> Derivative/1, Sum/1
  q/1 -> Sum/2
  Sum/1 -> lambda/1
  lambda/1 -> Sum1/2
  Sum1/1 -> qdotr/1
  Derivative/1 -> Sum1/1

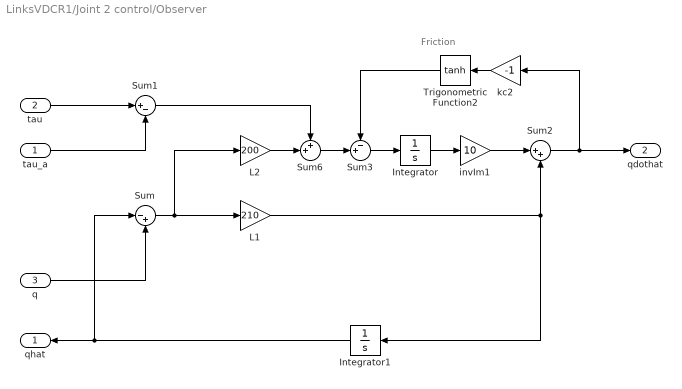
== system LinksVDCR1/Joint 2 control/Observer ==
  note: Friction
  tau_a : Inport
  tau : Inport  Port=2
  q : Inport  Port=3
  Integrator : Integrator
  Integrator1 : Integrator
  L1 : Gain  Gain=210
  L2 : Gain  Gain=200
  Sum : Sum  Inputs=|-+
  Sum1 : Sum  Inputs=|+-
  Sum2 : Sum  Inputs=|++
  Sum3 : Sum  Inputs=-+|
  Sum6 : Sum  Inputs=++|
  Trigonometric Function2 : Trigonometry  Operator=tanh
  invIm1 : Gain  Gain=10
  kc2 : Gain  Gain=-1
  qhat : Outport  VectorParamsAs1DForOutWhenUnconnected=off
  qdothat : Outport  Port=2  VectorParamsAs1DForOutWhenUnconnected=off
  wires:
  tau_a/1 -> Sum1/2
  tau/1 -> Sum1/1
  Sum/1 -> L2/1, L1/1
  q/1 -> Sum/2
  Sum1/1 -> Sum6/1
  L2/1 -> Sum6/2
  Integrator1/1 -> Sum/1, qhat/1
  Sum6/1 -> Sum3/2
  kc2/1 -> Trigonometric Function2/1
  Trigonometric Function2/1 -> Sum3/1
  Sum3/1 -> Integrator/1
  L1/1 -> Sum2/2, Integrator1/1
  Integrator/1 -> invIm1/1
  invIm1/1 -> Sum2/1
  Sum2/1 -> kc2/1, qdothat/1

== system LinksVDCR1/Joint 2 control/required ==
  q : Inport
  qd : Inport  Port=2
  Derivative : Derivative
  Sum : Sum  Inputs=+-|
  Sum1 : Sum  Inputs=++|
  lambda : Gain  Gain=10
  qdotr : Outport  VectorParamsAs1DForOutWhenUnconnected=off
  wires:
  qd/1 -> Derivative/1, Sum/1
  q/1 -> Sum/2
  Sum/1 -> lambda/1
  lambda/1 -> Sum1/2
  Sum1/1 -> qdotr/1
  Derivative/1 -> Sum1/1

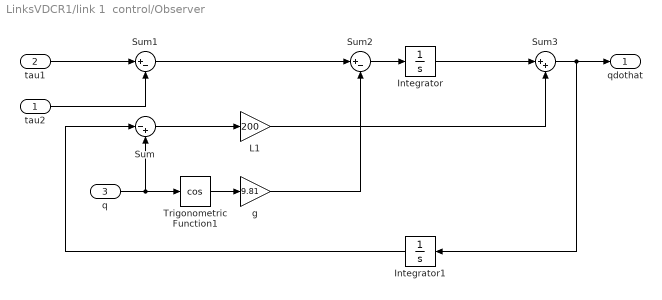
== system LinksVDCR1/link 1  control/Observer ==
  tau2 : Inport
  tau1 : Inport  Port=2
  q : Inport  Port=3
  Integrator : Integrator
  Integrator1 : Integrator
  L1 : Gain  Gain=200
  Sum : Sum  Inputs=|-+
  Sum1 : Sum  Inputs=|+-
  Sum2 : Sum  Inputs=|+-
  Sum3 : Sum  Inputs=|++
  Trigonometric Function1 : Trigonometry  Operator=cos
  g : Gain  Gain=9.81
  qdothat : Outport  VectorParamsAs1DForOutWhenUnconnected=off
  wires:
  tau2/1 -> Sum1/2
  tau1/1 -> Sum1/1
  Sum/1 -> L1/1
  Trigonometric Function1/1 -> g/1
  q/1 -> Trigonometric Function1/1, Sum/2
  g/1 -> Sum2/2
  Sum2/1 -> Integrator/1
  L1/1 -> Sum3/2
  Integrator1/1 -> Sum/1
  Sum1/1 -> Sum2/1
  Sum3/1 -> Integrator1/1, qdothat/1
  Integrator/1 -> Sum3/1

== matlab function LinksVDCR1/Link 2 observer/MATLAB Function2 ==
  data: q1 input; q2 input; P output
function P = fcn(q1, q2)

P = [sin(q1); cos(q1); q1 + q2];

== matlab function LinksVDCR1/Link 2 control/Fr ==
  data: Fin input; out output; g input
function out = fcn(Fin, g)
out = Fin + [0; 0; 1]*g;
end

== matlab function LinksVDCR1/Link 2 observer/Coriolis ==
  data: V input; Fc output
function Fc = fcn(V)

C = [0 -1 -1;1 0 0;1 0 0]*V(3);

Fc = C*V;

== matlab function LinksVDCR1/Link 2 control/Coriolis ==
  data: V input; Fc output; Vr input
function Fc = fcn(V, Vr)

C = [0 -1 -1;1 0 0;1 0 0]*V(3);

Fc = C*Vr;

== matlab function LinksVDCR1/Link 2 observer/MATLAB Function1 ==
  data: q2 input; V2 input; q1dot input; V output; q2dot output
function [V, q2dot] = fcn(q2, V2, q1dot)

q2dot = V2(3) - q1dot; 

V = [0 0 1]'*q2dot + [sin(q2); cos(q2); 1]*q1dot;

== matlab function LinksVDCR1/Link 2 control/F(3) ==
  data: in input; out output
function out = fcn(in)
out = in(3);

== matlab function LinksVDCR1/link 1  control/MATLAB Function ==
  data: F2r input; q1 input; q2 input; tau2r output
function tau2r = fcn(F2r, q1, q2)

tau2r = [sin(q2) cos(q2) 1]*F2r + 9.81*cos(q1);
% the last term has to do with gravity but it may belong elsewhere

== matlab function LinksVDCR1/Link 2 observer/required 2 ==
  data: q2 input; qdot2r input; qdot1r input; Vr output
function Vr = fcn(q2, qdot2r, qdot1r)

Vr = [0; 0; 1]*qdot2r + [sin(q2); cos(q2); 1]*qdot1r;
